simulink model "Controller"  (R2019b)
settings: Solver=VariableStepAuto  StartTime=0.0  StopTime=200  RelTol=1e-9
undefined symbols (not defined in the file or in its folder): D0, E0, I0, J0, R0, S0
libraries: simulink x3
settings Model: Creator=felipeareces  LastModifiedBy=felipeareces

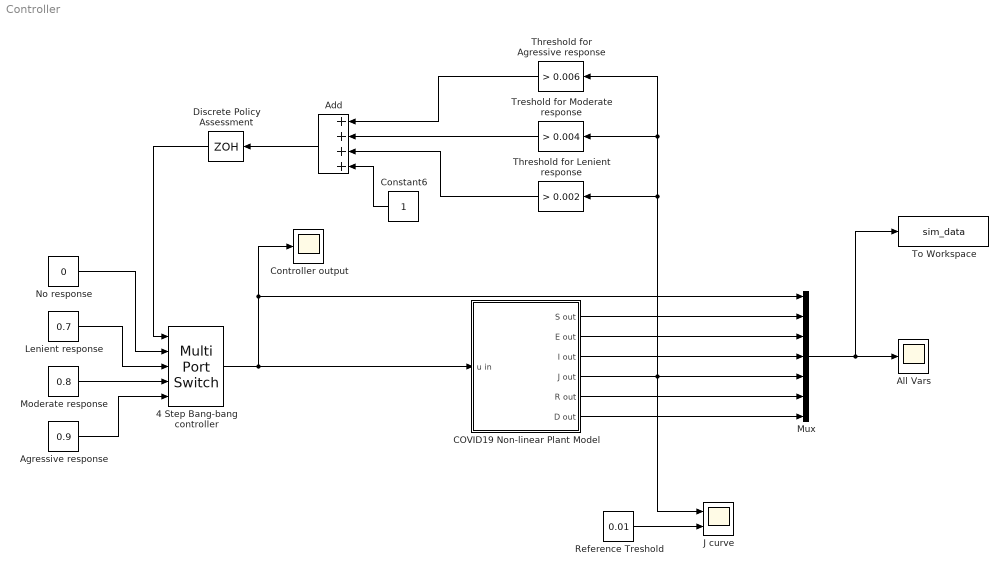
== system Controller ==
  4 Step Bang-bang controller : MultiPortSwitch  Inputs=4
  Add : Sum  Inputs=++++
  Agressive response : Constant  Value=0.9
  All Vars : Scope
  COVID19 Non-linear Plant Model : Subsystem
  Constant6 : Constant
  Controller output : Scope
  Discrete Policy Assessment : ZeroOrderHold  SampleTime=21
  J curve : Scope  NumInputPorts=2
  Lenient response : Constant  Value=0.7
  Moderate response : Constant  Value=0.8
  Mux : Mux  Inputs=7
  No response : Constant  Value=0
  Reference Treshold : Constant  Value=0.01
  Threshold for Agressive response : simulink/Logic and Bit Operations/Compare To Constant  relop=>  const=0.006  OutDataTypeStr=boolean
  Threshold for Lenient response : simulink/Logic and Bit Operations/Compare To Constant  relop=>  const=0.002  OutDataTypeStr=boolean
  To Workspace : ToWorkspace  VariableName=sim_data  SaveFormat=Timeseries  SampleTime=-1
  Treshold for Moderate response : simulink/Logic and Bit Operations/Compare To Constant  relop=>  const=0.004  OutDataTypeStr=boolean
  wires:
  COVID19 Non-linear Plant Model/4(J out) -> Treshold for Moderate response/1, Threshold for Agressive response/1, Threshold for Lenient response/1, Mux/5, J curve/1
  4 Step Bang-bang controller/1 -> COVID19 Non-linear Plant Model/1(u in), Controller output/1, Mux/1
  Threshold for Lenient response/1 -> Add/3
  Treshold for Moderate response/1 -> Add/2
  Threshold for Agressive response/1 -> Add/1
  Agressive response/1 -> 4 Step Bang-bang controller/5
  Moderate response/1 -> 4 Step Bang-bang controller/4
  Lenient response/1 -> 4 Step Bang-bang controller/3
  No response/1 -> 4 Step Bang-bang controller/2
  Constant6/1 -> Add/4
  Add/1 -> Discrete Policy Assessment/1
  Discrete Policy Assessment/1 -> 4 Step Bang-bang controller/1
  Reference Treshold/1 -> J curve/2
  COVID19 Non-linear Plant Model/1(S out) -> Mux/2
  COVID19 Non-linear Plant Model/2(E out) -> Mux/3
  COVID19 Non-linear Plant Model/3(I out) -> Mux/4
  COVID19 Non-linear Plant Model/5(R out) -> Mux/6
  COVID19 Non-linear Plant Model/6(D out) -> Mux/7
  Mux/1 -> All Vars/1, To Workspace/1

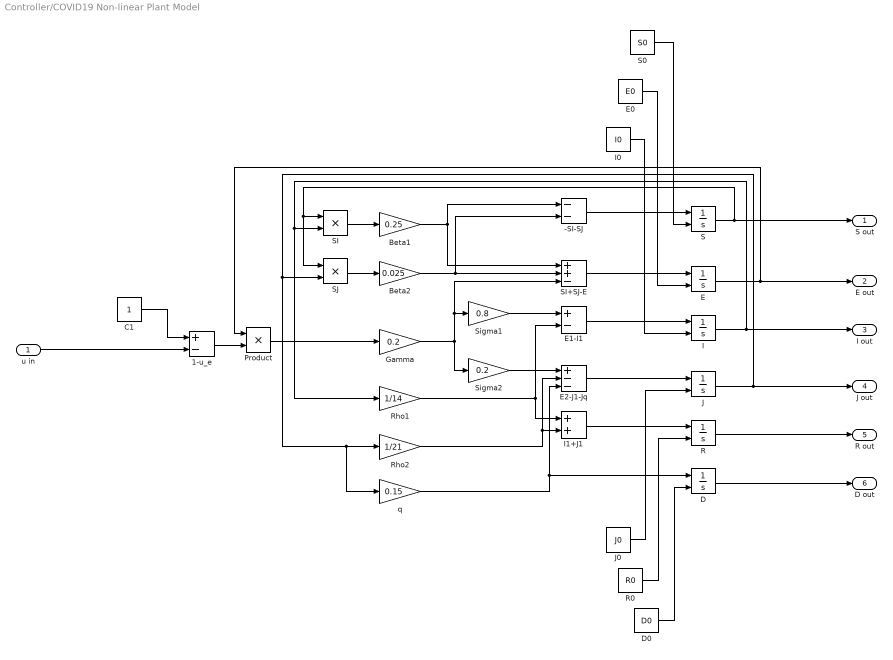
== system Controller/COVID19 Non-linear Plant Model ==
  u in : Inport
  -SI-SJ : Sum  Inputs=--
  1-u_e : Sum  Inputs=+-
  Beta1 : Gain  Gain=0.25
  Beta2 : Gain  Gain=0.025
  C1 : Constant
  D : Integrator  InitialConditionSource=external
  D0 : Constant  Value=D0
  E : Integrator  InitialConditionSource=external
  E0 : Constant  Value=E0
  E1-I1 : Sum  Inputs=+-
  E2-J1-Jq : Sum  Inputs=+--
  Gamma : Gain  Gain=0.2
  I : Integrator  InitialConditionSource=external
  I0 : Constant  Value=I0
  I1+J1 : Sum
  J : Integrator  InitialConditionSource=external
  J0 : Constant  Value=J0
  Product : Product
  R : Integrator  InitialConditionSource=external
  R0 : Constant  Value=R0
  Rho1 : Gain  Gain=1/14
  Rho2 : Gain  Gain=1/21
  S : Integrator  InitialConditionSource=external
  S0 : Constant  Value=S0
  SI : Product
  SI+SJ-E : Sum  Inputs=++-
  SJ : Product
  Sigma1 : Gain  Gain=0.8
  Sigma2 : Gain  Gain=0.2
  q : Gain  Gain=0.15
  S out : Outport
  E out : Outport  Port=2
  I out : Outport  Port=3
  J out : Outport  Port=4
  R out : Outport  Port=5
  D out : Outport  Port=6
  wires:
  u in/1 -> 1-u_e/2
  E2-J1-Jq/1 -> J/1
  R0/1 -> R/2
  Sigma2/1 -> E2-J1-Jq/1
  SI+SJ-E/1 -> E/1
  1-u_e/1 -> Product/2
  S/1 -> S out/1, SJ/1, SI/1
  I/1 -> I out/1, Rho1/1, SI/2
  Beta2/1 -> -SI-SJ/2, SI+SJ-E/2
  C1/1 -> 1-u_e/1
  D/1 -> D out/1
  E0/1 -> E/2
  Beta1/1 -> SI+SJ-E/1, -SI-SJ/1
  Gamma/1 -> Sigma2/1, SI+SJ-E/3, Sigma1/1
  q/1 -> E2-J1-Jq/3, D/1
  E/1 -> E out/1, Product/1
  J0/1 -> J/2
  S0/1 -> S/2
  Rho2/1 -> E2-J1-Jq/2, I1+J1/2
  E1-I1/1 -> I/1
  D0/1 -> D/2
  R/1 -> R out/1
  SJ/1 -> Beta2/1
  Product/1 -> Gamma/1
  I0/1 -> I/2
  Sigma1/1 -> E1-I1/1
  SI/1 -> Beta1/1
  -SI-SJ/1 -> S/1
  I1+J1/1 -> R/1
  Rho1/1 -> E1-I1/2, I1+J1/1
  J/1 -> q/1, Rho2/1, SJ/2, J out/1
